simulink model "flexible_drive"  (Simulink 8.7)
settings: Solver=ode45  StartTime=0.0  StopTime=9  RelTol=1e-3
values from neighbouring files (symbols this model uses):
  b1 = 0.0097    [q1_2.m]
  b2 = 0.00097122    [q1_2.m]
  d1 = 0.793    [q1_2.m]
  d2 = 0.0793    [q1_2.m]
  k = 0.0466    [q1_2.m]
  m1 = 0.00031218    [q1_2.m]
  m2 = 0.00016858    [q1_2.m]
undefined symbols (not defined in the file or in its folder): c, sgn, Ts
settings Model: Creator=user  LastModifiedBy=user
settings DataIOCC: SignalLoggingSaveFormat=ModelDataLogs  SignalLoggingName=sigsOut
settings DebuggingCC: SaveWithParameterizedLinksMsg=none  SignalResolutionControl=TryResolveAllWithWarning  MultiTaskDSMMsg=warning  MultiTaskCondExecSysMsg=none
settings HardwareCC: TargetUnknown=on
settings GRTTargetCC: GeneratePreprocessorConditionals=Use local settings  CombineOutputUpdateFcns=off  GRTInterface=on

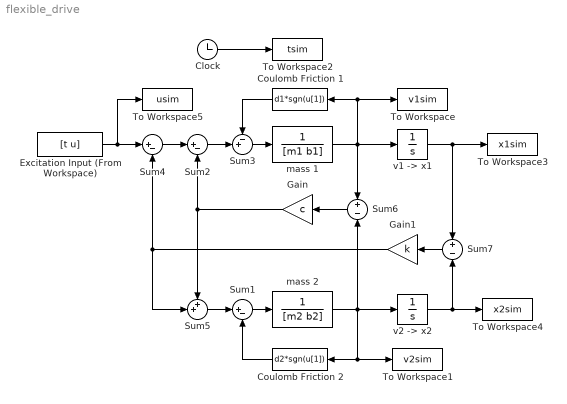
== system flexible_drive ==
  Clock : Clock
  Coulomb Friction 1 : Fcn  Expr=d1*sgn(u[1])
  Coulomb Friction 2 : Fcn  Expr=d2*sgn(u[1])
  Excitation Input (From Workspace) : FromWorkspace  VariableName=[t u]  SampleTime=Ts  OutputAfterFinalValue=Holding final value
  Gain : Gain  Gain=c  SaturateOnIntegerOverflow=on  OutDataTypeStr=Inherit: Same as input  ParamDataTypeStr=Inherit: Same as input
  Gain1 : Gain  Gain=k  SaturateOnIntegerOverflow=on  OutDataTypeStr=Inherit: Same as input  ParamDataTypeStr=Inherit: Same as input
  Sum1 : Sum  Inputs=|+-  SaturateOnIntegerOverflow=on
  Sum2 : Sum  Inputs=|+-  SaturateOnIntegerOverflow=on
  Sum3 : Sum  Inputs=-+|  SaturateOnIntegerOverflow=on
  Sum4 : Sum  Inputs=|+-  SaturateOnIntegerOverflow=on
  Sum5 : Sum  Inputs=++|  SaturateOnIntegerOverflow=on
  Sum6 : Sum  Inputs=+|-  SaturateOnIntegerOverflow=on
  Sum7 : Sum  Inputs=+|-  SaturateOnIntegerOverflow=on
  To Workspace : ToWorkspace  VariableName=v1sim  SampleTime=Ts
  To Workspace1 : ToWorkspace  VariableName=v2sim  SampleTime=Ts
  To Workspace2 : ToWorkspace  VariableName=tsim  SampleTime=Ts
  To Workspace3 : ToWorkspace  VariableName=x1sim  SampleTime=Ts
  To Workspace4 : ToWorkspace  VariableName=x2sim  SampleTime=Ts
  To Workspace5 : ToWorkspace  VariableName=usim  SampleTime=Ts
  mass 1 : TransferFcn  Denominator=[m1 b1]
  mass 2 : TransferFcn  Denominator=[m2 b2]
  "v1 -> x1" : Integrator
  "v2 -> x2" : Integrator
  wires:
  mass 1/1 -> "v1 -> x1"/1, Sum6/1, Coulomb Friction 1/1, To Workspace/1
  Clock/1 -> To Workspace2/1
  Sum3/1 -> mass 1/1
  Coulomb Friction 1/1 -> Sum3/1
  mass 2/1 -> "v2 -> x2"/1, Sum6/2, Coulomb Friction 2/1, To Workspace1/1
  Sum1/1 -> mass 2/1
  Coulomb Friction 2/1 -> Sum1/2
  Sum2/1 -> Sum3/2
  Sum5/1 -> Sum1/1
  Sum6/1 -> Gain/1
  Gain/1 -> Sum2/2, Sum5/1
  "v1 -> x1"/1 -> Sum7/1, To Workspace3/1
  "v2 -> x2"/1 -> Sum7/2, To Workspace4/1
  Sum7/1 -> Gain1/1
  Gain1/1 -> Sum4/2, Sum5/2
  Sum4/1 -> Sum2/1
  Excitation Input (From Workspace)/1 -> Sum4/1, To Workspace5/1
